simulink model "day07"  (R2026a)
settings: Solver=VariableStepAuto  StopTime=inf
undefined symbols (not defined in the file): DiscIntNeverNeededParam
libraries: simulink x4
settings Model: Creator=pete  LastModifiedBy=pete

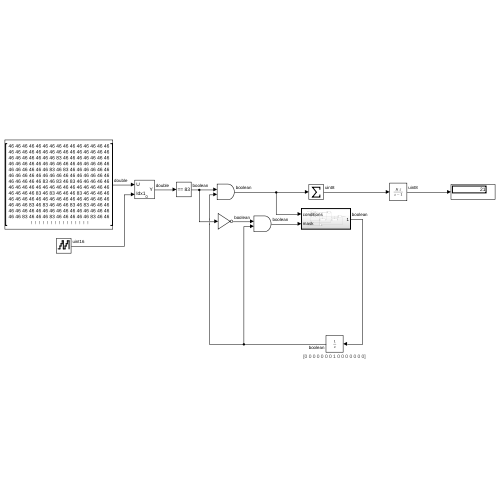
[thumbnail: Simulink's stored preview of the top-level diagram]
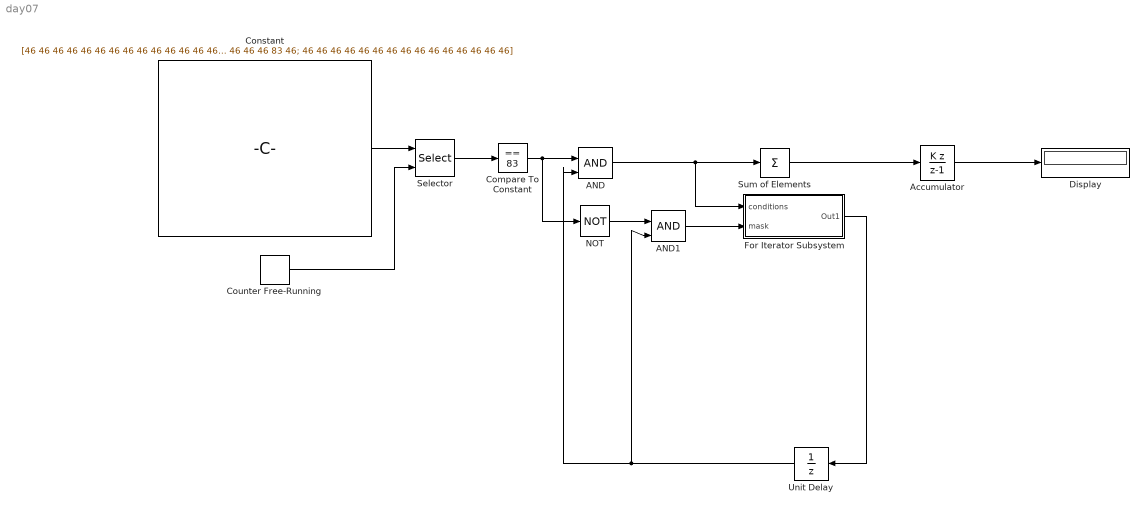
== system day07 ==
  AND : Logic  IconShape=distinctive  AllPortsSameDT=off  OutDataTypeStr=boolean
  AND1 : Logic  IconShape=distinctive  AllPortsSameDT=off  OutDataTypeStr=boolean
  Accumulator : DiscreteIntegrator  IntegratorMethod=Accumulation: Backward Euler  SampleTime=-1  ICPrevOutput=DiscIntNeverNeededParam  ICPrevScaledInput=DiscIntNeverNeededParam
  Compare To Constant : simulink/Logic and Bit Operations/Compare To Constant  relop===  const=83  OutDataTypeStr=boolean
  Constant : Constant  Value=|
      | [46 46 46 46 46 46 46 46 46 46 46 46 46 46 46;
      | 46 46 46 46 46 46 46 46 46 46 46 46 46 46 46;
      | 46 46 46 46 46 46 46 83 46 46 46 46 46 46 46;
      | 46 46 46 46 46 46 46 46 46 46 46 46 46 46 46;
      | 46 46 46 46 46 46 83 46 83 46 46 46 46 46 46;
      | 46 46 46 46 46 46 46 46 46 46 46 46 46 46 46;
      | 46 46 46 46 46 83 46 83 46 83 46 46 46 46 46;
      | 46 46 46 46 46 46 46 46 46 46 46 46 46 46 46;
      | 46 46 46 46 83 46 83 46 46 46 83 46 46 46 46;
      | 46 46 46 46 46 46 46 46 46 46 46 46 46 46 46;
      | 46 46 46 83 46 83 46 46 46 83 46 83 46 46 46;
      | 46 46 46 46 46 46 46 46 46 46 46 46 46 46 46;
      | 46 46 83 46 46 46 83 46 46 46 46 46 83 46 46;
      | 46 46 46 46 46 46 46 46 46 46 46 46 46 46 46;
      | 46 83 46 83 46 83 46 83 46 83 46 46 46 83 46;
      | 46 46 46 46 46 46 46 46 46 46 46 46 46 46 46]
  Counter Free-Running : simulink/Sources/Counter Free-Running  NumBits=16  tsamp=-1
  Display : Display
  For Iterator Subsystem : Subsystem  TreatAsAtomicUnit=on
  NOT : Logic  Operator=NOT  IconShape=distinctive  AllPortsSameDT=off  OutDataTypeStr=boolean
  Selector : Selector  NumberOfDimensions=2  IndexMode=Zero-based  InputPortWidth=3  IndexOptions=Index vector (port),Index vector (dialog)  Indices=[1 3],[0:14]  OutputSizes=1,1
  Sum of Elements : Sum  Inputs=+
  Unit Delay : UnitDelay  InitialCondition=[0 0 0 0 0 0 0 1 0 0 0 0 0 0 0]  SampleTime=-1
      settings: AttributesFormatString=%<InitialCondition>
  wires:
  Constant/1 -> Selector/1
  Counter Free-Running/1 -> Selector/2
  Selector/1 -> Compare To Constant/1
  Compare To Constant/1 -> NOT/1, AND/1
  Unit Delay/1 -> AND/2, AND1/2
  NOT/1 -> AND1/1
  AND/1 -> For Iterator Subsystem/1(conditions), Sum of Elements/1
  Sum of Elements/1 -> Accumulator/1
  Accumulator/1 -> Display/1
  AND1/1 -> For Iterator Subsystem/2(mask)
  For Iterator Subsystem/1(Out1) -> Unit Delay/1

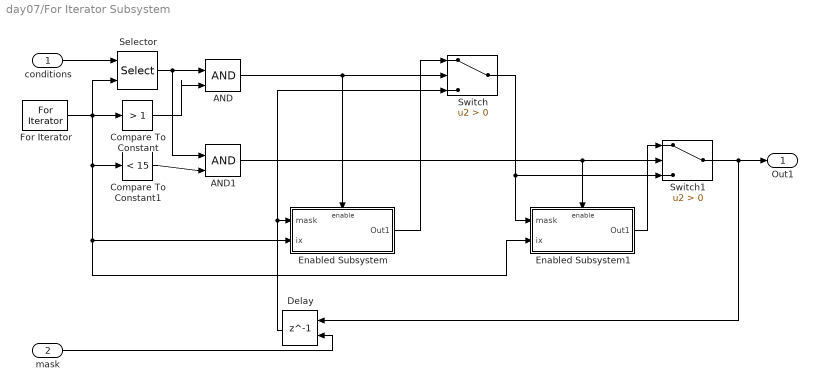
== system day07/For Iterator Subsystem ==
  conditions : Inport
  mask : Inport  Port=2
  AND : Logic  IconShape=distinctive  AllPortsSameDT=off  OutDataTypeStr=boolean
  AND1 : Logic  IconShape=distinctive  AllPortsSameDT=off  OutDataTypeStr=boolean
  Compare To Constant : simulink/Logic and Bit Operations/Compare To Constant  relop=>  const=1  OutDataTypeStr=boolean
  Compare To Constant1 : simulink/Logic and Bit Operations/Compare To Constant  relop=<  const=15  OutDataTypeStr=boolean
  Delay : Delay  DelayLength=1  InitialConditionSource=Input port
      settings: InputPortMap=u0,p4
  Enabled Subsystem : Subsystem  TreatAsAtomicUnit=on
  Enabled Subsystem1 : Subsystem  TreatAsAtomicUnit=on
  For Iterator : ForIterator  ResetStates=reset  IterationLimit=15
      settings: AttributesFormatString=|
      | %<IterationLimit>
      | %<ResetStates>
  Selector : Selector  InputPortWidth=15  IndexOptions=Index vector (port)  Indices=[1 3]  OutputSizes=1
  Switch : Switch  Criteria=u2 > Threshold  SaturateOnIntegerOverflow=off  InputSameDT=off
  Switch1 : Switch  Criteria=u2 > Threshold  SaturateOnIntegerOverflow=off  InputSameDT=off
  Out1 : Outport
  wires:
  conditions/1 -> Selector/1
  For Iterator/1 -> Enabled Subsystem1/2(ix), Enabled Subsystem/2(ix), Compare To Constant1/1, Compare To Constant/1, Selector/2
  Selector/1 -> AND1/1, AND/1
  Compare To Constant/1 -> AND/2
  Compare To Constant1/1 -> AND1/2
  mask/1 -> Delay/2
  Delay/1 -> Switch/3, Enabled Subsystem/1(mask)
  AND/1 -> Switch/2, Enabled Subsystem/Enable
  Enabled Subsystem/1(Out1) -> Switch/1
  Switch/1 -> Switch1/3, Enabled Subsystem1/1(mask)
  AND1/1 -> Switch1/2, Enabled Subsystem1/Enable
  Enabled Subsystem1/1(Out1) -> Switch1/1
  Switch1/1 -> Delay/1, Out1/1

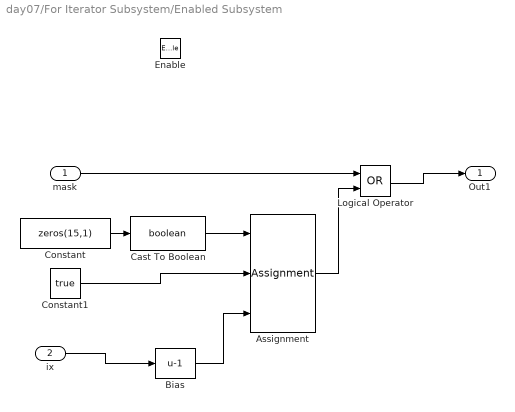
== system day07/For Iterator Subsystem/Enabled Subsystem ==
  mask : Inport
  ix : Inport  Port=2
  Enable : EnablePort
  Assignment : Assignment  DiagnosticForDimensions=Warning  IndexOptions=Index vector (port)  Indices=1  OutputSizes=1
  Bias : Bias  Bias=-1  SaturateOnIntegerOverflow=off
  Cast To Boolean : DataTypeConversion  OutDataTypeStr=boolean  SaturateOnIntegerOverflow=off  RndMeth=Floor
  Constant : Constant  Value=zeros(15,1)
  Constant1 : Constant  Value=true
  Logical Operator : Logic  Operator=OR  AllPortsSameDT=off  OutDataTypeStr=boolean
  Out1 : Outport
  wires:
  Constant/1 -> Cast To Boolean/1
  ix/1 -> Bias/1
  Cast To Boolean/1 -> Assignment/1
  Constant1/1 -> Assignment/2
  Bias/1 -> Assignment/3
  mask/1 -> Logical Operator/1
  Assignment/1 -> Logical Operator/2
  Logical Operator/1 -> Out1/1

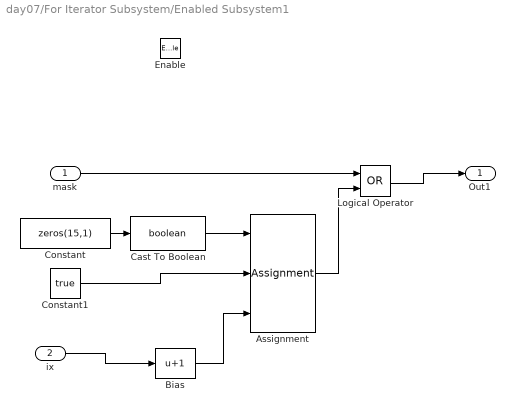
== system day07/For Iterator Subsystem/Enabled Subsystem1 ==
  mask : Inport
  ix : Inport  Port=2
  Enable : EnablePort
  Assignment : Assignment  DiagnosticForDimensions=Warning  IndexOptions=Index vector (port)  Indices=1  OutputSizes=1
  Bias : Bias  Bias=1  SaturateOnIntegerOverflow=off
  Cast To Boolean : DataTypeConversion  OutDataTypeStr=boolean  SaturateOnIntegerOverflow=off  RndMeth=Floor
  Constant : Constant  Value=zeros(15,1)
  Constant1 : Constant  Value=true
  Logical Operator : Logic  Operator=OR  AllPortsSameDT=off  OutDataTypeStr=boolean
  Out1 : Outport
  wires:
  Constant/1 -> Cast To Boolean/1
  ix/1 -> Bias/1
  Cast To Boolean/1 -> Assignment/1
  Constant1/1 -> Assignment/2
  Bias/1 -> Assignment/3
  mask/1 -> Logical Operator/1
  Assignment/1 -> Logical Operator/2
  Logical Operator/1 -> Out1/1
